simulink model "quad_3_ref_NN"  (R2018b)
settings: Solver=VariableStepAuto  StartTime=0.0  StopTime=20  RelTol=1e-3
undefined symbols (not defined in the file or in its folder): options
libraries: neural x70, simulink x3
(part 2 of 4)

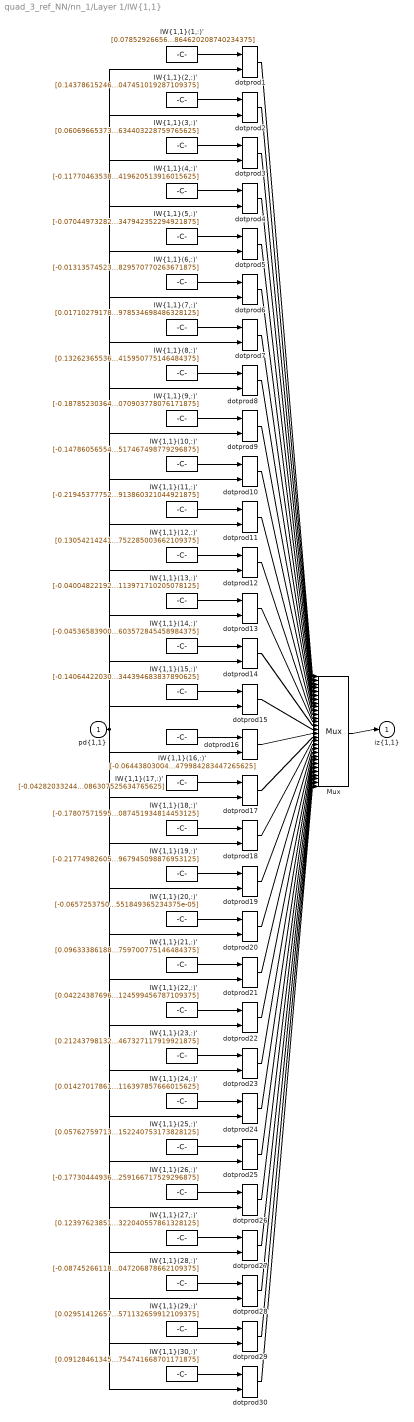
== system quad_3_ref_NN/nn_1/Layer 1/IW{1,1} ==
  "pd{1,1}" : Inport  PortDimensions=12
      mask Display: e = 0.06;c1 = [120 230 180]/255;c2 = ([120 230 180]+0)/(256+128);c3 = ([120 230 180]+128)/(256+128);patch([0 1 1 0],[0 0 1 1],c1);patch([0 1 1 1-e 1-e 0+e],[0 0 1 1-e 0+e 0+e],c2);patch([0 0 1 1-e 0+e 0+e],[0 1 1 1-e 1-e 0+e],c3);plot([0 1 1 0 0],[0 0 1 1 0]);
  "IW{1,1}(1,:)'" : Constant  Value=[0.078529266562737121137871554310549981892108917236328125;0.00786693915550643572964784056011922075413167476654052734375;0.002443768882647874736424586927796553936786949634552001953125;-0.07263690237927265813677735195597051642835140228271484375;0.01107188552850253519810319602356685209088027477264404296875;-0.0207620276565758342390832780210985220037400722503662109375;0.0370645742360258545478046698917751200497150421142578125;0.0256582074103387063057635231189124169759452342987060546875;0.00430276640258473765110469599903808557428419589996337890625;-0.0037272719818124311515206148470724656363017857074737548828125;0.0142728984479785735162149507004869519732892513275146484375;0.01071616499854453029294543142668771906755864620208740234375]
      mask Display: e = 0.06;c1 = [120 150 230]/255;c2 = ([120 150 230]+0)/383;c3 = ([120 150 230]+128)/383;patch([0 1 1 0],[0 0 1 1],c1);patch([0 1 1 1-e 1-e 0+e],[0 0 1 1-e 0+e 0+e],c2);patch([0 0 1 1-e 0+e 0+e],[0 1 1 1-e 1-e 0+e],c3);plot([0 1 1 0 0],[0 0 1 1 0]);disp('Weights');
  "IW{1,1}(10,:)'" : Constant  Value=[-0.147860565541055366534095583119778893887996673583984375;0.0134470182788290378017581616632014629431068897247314453125;-0.0040992668073650852245126685602372162975370883941650390625;0.2037966130921315954793726632487960159778594970703125;-0.02318330531982816522518220381243736483156681060791015625;0.00827620039422155388819657417798225651495158672332763671875;-0.03711045306748207706082354206955642439424991607666015625;-0.010840372744474746635745532330474816262722015380859375;-0.0160737259669415342988596506756948656402528285980224609375;0.005420268773988205779357230085224728100001811981201171875;0.01523382841408883747735814040424884296953678131103515625;0.0193009061476432479398379626900350558571517467498779296875]
      mask Display: e = 0.06;c1 = [120 150 230]/255;c2 = ([120 150 230]+0)/383;c3 = ([120 150 230]+128)/383;patch([0 1 1 0],[0 0 1 1],c1);patch([0 1 1 1-e 1-e 0+e],[0 0 1 1-e 0+e 0+e],c2);patch([0 0 1 1-e 0+e 0+e],[0 1 1 1-e 1-e 0+e],c3);plot([0 1 1 0 0],[0 0 1 1 0]);disp('Weights');
  "IW{1,1}(11,:)'" : Constant  Value=[-0.21945377752996531039997307743760757148265838623046875;0.026810922938275104365768441994077875278890132904052734375;0.0216877503417858934209316856822624686174094676971435546875;0.352460566654302864808556705611408688127994537353515625;0.0480097492404133185939230088479234836995601654052734375;-0.017400965439232397857782785877134301699697971343994140625;-0.134722352421196400751313149157795123755931854248046875;0.028292010630161616713262873190615209750831127166748046875;0.040633554867679867739216348354602814652025699615478515625;0.030043134050046362004682265478550107218325138092041015625;0.03901470178400827382159121725635486654937267303466796875;0.0600659941011620623907418803355540148913860321044921875]
      mask Display: e = 0.06;c1 = [120 150 230]/255;c2 = ([120 150 230]+0)/383;c3 = ([120 150 230]+128)/383;patch([0 1 1 0],[0 0 1 1],c1);patch([0 1 1 1-e 1-e 0+e],[0 0 1 1-e 0+e 0+e],c2);patch([0 0 1 1-e 0+e 0+e],[0 1 1 1-e 1-e 0+e],c3);plot([0 1 1 0 0],[0 0 1 1 0]);disp('Weights');
  "IW{1,1}(12,:)'" : Constant  Value=[0.13054214241561179488115840285900048911571502685546875;-0.010876253958645880348665713199807214550673961639404296875;0.00645744195837419897310294203407465829513967037200927734375;-0.1590334124757807610084370253389352001249790191650390625;0.003502550214369952452653222962908330373466014862060546875;-0.0177574896271106286160801346341031603515148162841796875;0.0307044845016924451697182263387730927206575870513916015625;0.0198496171972888969803339165309807867743074893951416015625;0.0165141943466253805772314677824397222138941287994384765625;-0.008272558443627182900304006807346013374626636505126953125;-0.016577272283062348401383445661849691532552242279052734375;-0.019815470714216541769925328253521001897752285003662109375]
      mask Display: e = 0.06;c1 = [120 150 230]/255;c2 = ([120 150 230]+0)/383;c3 = ([120 150 230]+128)/383;patch([0 1 1 0],[0 0 1 1],c1);patch([0 1 1 1-e 1-e 0+e],[0 0 1 1-e 0+e 0+e],c2);patch([0 0 1 1-e 0+e 0+e],[0 1 1 1-e 1-e 0+e],c3);plot([0 1 1 0 0],[0 0 1 1 0]);disp('Weights');
  "IW{1,1}(13,:)'" : Constant  Value=[-0.0400482219240929915304860742253367789089679718017578125;-0.01136951268733107749120403440201698685996234416961669921875;-0.01275137584911217349115108987689382047392427921295166015625;0.019746638647258070442536137534261797554790973663330078125;-0.0100133008805152988462960905735599226318299770355224609375;0.00554886997693828688815731453587432042695581912994384765625;-0.0207279164856813795381196285916303168050944805145263671875;-0.0132145956485405884073269788814286584965884685516357421875;-0.0154206941241152480082110542980444733984768390655517578125;-0.0017440958504595879298426641668129377649165689945220947265625;-0.0118417785038119893759045453407452441751956939697265625;-0.0003297525368371159899816280614004426752217113971710205078125]
      mask Display: e = 0.06;c1 = [120 150 230]/255;c2 = ([120 150 230]+0)/383;c3 = ([120 150 230]+128)/383;patch([0 1 1 0],[0 0 1 1],c1);patch([0 1 1 1-e 1-e 0+e],[0 0 1 1-e 0+e 0+e],c2);patch([0 0 1 1-e 0+e 0+e],[0 1 1 1-e 1-e 0+e],c3);plot([0 1 1 0 0],[0 0 1 1 0]);disp('Weights');
  "IW{1,1}(14,:)'" : Constant  Value=[-0.04536583900623207543656434381773578934371471405029296875;0.015322325707905641578587818685264210216701030731201171875;0.016285107900788527157676099932359647937119007110595703125;0.01209169860414867347930822916168835945427417755126953125;-0.009840496063433755435934102706596604548394680023193359375;-0.001097090523768812393712313024707327713258564472198486328125;0.00288142231145414873250132359316921792924404144287109375;0.000899839764804431958833408344844428938813507556915283203125;-0.00132219817163032292428592739952364354394376277923583984375;0.01485548166720073066937590766656285268254578113555908203125;0.00875988621009281265283874517990625463426113128662109375;0.00159143009482582385716309403278501122258603572845458984375]
      mask Display: e = 0.06;c1 = [120 150 230]/255;c2 = ([120 150 230]+0)/383;c3 = ([120 150 230]+128)/383;patch([0 1 1 0],[0 0 1 1],c1);patch([0 1 1 1-e 1-e 0+e],[0 0 1 1-e 0+e 0+e],c2);patch([0 0 1 1-e 0+e 0+e],[0 1 1 1-e 1-e 0+e],c3);plot([0 1 1 0 0],[0 0 1 1 0]);disp('Weights');
  "IW{1,1}(15,:)'" : Constant  Value=[-0.1406442203035578042413789034981164149940013885498046875;-0.00489135033403387264883122043102048337459564208984375;-0.003944791983629051916604435490398827823810279369354248046875;0.1445432054926384657367322006393806077539920806884765625;-0.0130691593280128637299952742978348396718502044677734375;0.01510921933796705897423695574843804934062063694000244140625;-0.08150926462194003907502093397852149792015552520751953125;0.00943571383983794580163628751279247808270156383514404296875;0.01004127751787367399394224065645175869576632976531982421875;-0.0183353986201333536698587778346336563117802143096923828125;-0.0157985391490613018283806212593844975344836711883544921875;-0.0161584671239796452690828942877487861551344394683837890625]
      mask Display: e = 0.06;c1 = [120 150 230]/255;c2 = ([120 150 230]+0)/383;c3 = ([120 150 230]+128)/383;patch([0 1 1 0],[0 0 1 1],c1);patch([0 1 1 1-e 1-e 0+e],[0 0 1 1-e 0+e 0+e],c2);patch([0 0 1 1-e 0+e 0+e],[0 1 1 1-e 1-e 0+e],c3);plot([0 1 1 0 0],[0 0 1 1 0]);disp('Weights');
  "IW{1,1}(16,:)'" : Constant  Value=[-0.0644380300412848161517587186608579941093921661376953125;0.001197491485301433768173584581973045715130865573883056640625;-0.002973574198419578172580823860471355146728456020355224609375;0.07261552598673505498627633869546116329729557037353515625;-0.00911983882616861606107416804434251389466226100921630859375;0.002258921289302671768506325378211840870790183544158935546875;-0.01497592283162310113076021167444196180440485477447509765625;0.00432259258477654152719171776197981671430170536041259765625;-0.01530863786152473517143679515584153705276548862457275390625;0.0011924005049313009078904013193778155255131423473358154296875;0.001075716311985324726008261819742983789183199405670166015625;-0.0180167069664866098810396266571842716075479984283447265625]
      mask Display: e = 0.06;c1 = [120 150 230]/255;c2 = ([120 150 230]+0)/383;c3 = ([120 150 230]+128)/383;patch([0 1 1 0],[0 0 1 1],c1);patch([0 1 1 1-e 1-e 0+e],[0 0 1 1-e 0+e 0+e],c2);patch([0 0 1 1-e 0+e 0+e],[0 1 1 1-e 1-e 0+e],c3);plot([0 1 1 0 0],[0 0 1 1 0]);disp('Weights');
  "IW{1,1}(17,:)'" : Constant  Value=[-0.042820332449136418173640805662216735072433948516845703125;-0.0065443141325867669466642695397240458987653255462646484375;-0.01513063676343030621029850379954950767569243907928466796875;0.032196066510549424533049744923118851147592067718505859375;-0.0033468345050003613268263524815893106278963387012481689453125;0.00461329995651396131128851862968076602555811405181884765625;-0.002691478208598889650116081639907861244864761829376220703125;0.000650547080040542353984722723225786467082798480987548828125;-0.01729420381033273945714512365157133899629116058349609375;0.00405337807023969064201818213177830330096185207366943359375;-0.01149323371723583175896266084237140603363513946533203125;-0.0045561415204842282966612998507116572000086307525634765625]
      mask Display: e = 0.06;c1 = [120 150 230]/255;c2 = ([120 150 230]+0)/383;c3 = ([120 150 230]+128)/383;patch([0 1 1 0],[0 0 1 1],c1);patch([0 1 1 1-e 1-e 0+e],[0 0 1 1-e 0+e 0+e],c2);patch([0 0 1 1-e 0+e 0+e],[0 1 1 1-e 1-e 0+e],c3);plot([0 1 1 0 0],[0 0 1 1 0]);disp('Weights');
  "IW{1,1}(18,:)'" : Constant  Value=[-0.1780757159575738768353403429500758647918701171875;-0.019521046281996905225053495769316214136779308319091796875;-0.02148481740437359344131351690521114505827426910400390625;0.2394798892014605995459675114034325815737247467041015625;0.020440374862543873868414578964802785776555538177490234375;-0.01235558398060544217644807218903224566020071506500244140625;-0.1228380733929725909803210015525110065937042236328125;0.0139497234295006093673929825627055834047496318817138671875;0.01213816245689446071676087512969388626515865325927734375;-0.033165603622792076687897377951230737380683422088623046875;-0.0269775987766404691525767844950678409077227115631103515625;-0.0084178593815306575198764704737186548300087451934814453125]
      mask Display: e = 0.06;c1 = [120 150 230]/255;c2 = ([120 150 230]+0)/383;c3 = ([120 150 230]+128)/383;patch([0 1 1 0],[0 0 1 1],c1);patch([0 1 1 1-e 1-e 0+e],[0 0 1 1-e 0+e 0+e],c2);patch([0 0 1 1-e 0+e 0+e],[0 1 1 1-e 1-e 0+e],c3);plot([0 1 1 0 0],[0 0 1 1 0]);disp('Weights');
  "IW{1,1}(19,:)'" : Constant  Value=[-0.2177498260504428240214025436216616071760654449462890625;0.0185045242913031461606809813247309648431837558746337890625;0.0016690905058854392517542208906888845376670360565185546875;0.25350570394707194754602141983923502266407012939453125;0.0080543188283483217737579451522833551280200481414794921875;-0.003408997157735411953627391312693362124264240264892578125;-0.1300658296282164172463780005273292772471904754638671875;0.0118027299680211437971077970132682821713387966156005859375;-0.009127017617710224406391006368721718899905681610107421875;0.00992258872258855451065073793870396912097930908203125;-0.000647670814953184292850352221648790873587131500244140625;-0.012919553810417212791339380828503635711967945098876953125]
      mask Display: e = 0.06;c1 = [120 150 230]/255;c2 = ([120 150 230]+0)/383;c3 = ([120 150 230]+128)/383;patch([0 1 1 0],[0 0 1 1],c1);patch([0 1 1 1-e 1-e 0+e],[0 0 1 1-e 0+e 0+e],c2);patch([0 0 1 1-e 0+e 0+e],[0 1 1 1-e 1-e 0+e],c3);plot([0 1 1 0 0],[0 0 1 1 0]);disp('Weights');
  "IW{1,1}(2,:)'" : Constant  Value=[0.1437861524654724387772830596077255904674530029296875;-0.004658330850192315443492052651208723546005785465240478515625;0.0166751004439475158935834997464553453028202056884765625;-0.163922574492781636390503763323067687451839447021484375;0.01526933862748157400002213535117334686219692230224609375;-0.00976544107933535916743483795698921312578022480010986328125;0.054240136556781330667842411230594734661281108856201171875;0.013842710387504543467773743259385810233652591705322265625;0.008788677192960343831362735045331646688282489776611328125;0.0143984192110828169985925484297695220448076725006103515625;0.02277789638211417944102521460081334225833415985107421875;0.018991406808802978323225119083872414194047451019287109375]
      mask Display: e = 0.06;c1 = [120 150 230]/255;c2 = ([120 150 230]+0)/383;c3 = ([120 150 230]+128)/383;patch([0 1 1 0],[0 0 1 1],c1);patch([0 1 1 1-e 1-e 0+e],[0 0 1 1-e 0+e 0+e],c2);patch([0 0 1 1-e 0+e 0+e],[0 1 1 1-e 1-e 0+e],c3);plot([0 1 1 0 0],[0 0 1 1 0]);disp('Weights');
  "IW{1,1}(20,:)'" : Constant  Value=[-0.06572537506185331668273619243336725048720836639404296875;0.01669642639971923026021016767117544077336788177490234375;0.01438697051899651656314826908555914997123181819915771484375;0.097990860021580694638743125324253924190998077392578125;-0.023250392969835768919306673296887311153113842010498046875;0.034191678885905997520300303449403145350515842437744140625;0.00207157777178058714884212321294398861937224864959716796875;-0.03102709202383165110195051283881184644997119903564453125;-0.02967893733167838166142615818898775614798069000244140625;0.01480263260132471010710464298654187587089836597442626953125;0.0152700053015788032861888012803319725207984447479248046875;-3.5242403931787756599103289545382722280919551849365234375e-05]
      mask Display: e = 0.06;c1 = [120 150 230]/255;c2 = ([120 150 230]+0)/383;c3 = ([120 150 230]+128)/383;patch([0 1 1 0],[0 0 1 1],c1);patch([0 1 1 1-e 1-e 0+e],[0 0 1 1-e 0+e 0+e],c2);patch([0 0 1 1-e 0+e 0+e],[0 1 1 1-e 1-e 0+e],c3);plot([0 1 1 0 0],[0 0 1 1 0]);disp('Weights');
  "IW{1,1}(21,:)'" : Constant  Value=[0.0963338618860876960692252168882987461984157562255859375;-0.017399790836133639804206296730626490898430347442626953125;-0.0190305406288347016274808964908515918068587779998779296875;-0.08916389166021602974421256249115685932338237762451171875;0.00790176839013517588738988450813849340192973613739013671875;-0.01478596274658084720743378426277558901347219944000244140625;0.0029569260110624100146292647650625440292060375213623046875;0.02925230114780884294045648630344658158719539642333984375;0.01150080739869995503921185076023903093300759792327880859375;-0.0173239132576814454378411056723052752204239368438720703125;-0.0251577527719447739673608310795316356234252452850341796875;-0.0284567136595101910501171005307696759700775146484375]
      mask Display: e = 0.06;c1 = [120 150 230]/255;c2 = ([120 150 230]+0)/383;c3 = ([120 150 230]+128)/383;patch([0 1 1 0],[0 0 1 1],c1);patch([0 1 1 1-e 1-e 0+e],[0 0 1 1-e 0+e 0+e],c2);patch([0 0 1 1-e 0+e 0+e],[0 1 1 1-e 1-e 0+e],c3);plot([0 1 1 0 0],[0 0 1 1 0]);disp('Weights');
  "IW{1,1}(22,:)'" : Constant  Value=[0.04224387696688165771963241468256455846130847930908203125;-0.0072788809324365842667869941351455054245889186859130859375;-0.00776694166044583807206880265994186629541218280792236328125;-0.039942992962429001158053409881176776252686977386474609375;-0.002529471782466141509260193487307333271019160747528076171875;2.276536562523766293875127075807540677487850189208984375e-05;0.004836203064547402001582820929570516454987227916717529296875;-0.00802404233775699630981659282724649528972804546356201171875;-0.0010166811297409139407121880793738455395214259624481201171875;-0.0021571010148963682372114103458216050057671964168548583984375;0.005758936473604313842356017261181477806530892848968505859375;-0.0109210797386651535523238720770677900873124599456787109375]
      mask Display: e = 0.06;c1 = [120 150 230]/255;c2 = ([120 150 230]+0)/383;c3 = ([120 150 230]+128)/383;patch([0 1 1 0],[0 0 1 1],c1);patch([0 1 1 1-e 1-e 0+e],[0 0 1 1-e 0+e 0+e],c2);patch([0 0 1 1-e 0+e 0+e],[0 1 1 1-e 1-e 0+e],c3);plot([0 1 1 0 0],[0 0 1 1 0]);disp('Weights');
  "IW{1,1}(23,:)'" : Constant  Value=[0.2124379813207072087433147089541307650506496429443359375;0.0271084126562651517300395198617479763925075531005859375;0.03617241440309056088597827738340129144489765167236328125;-0.2329129512256800371705622865192708559334278106689453125;-0.006326850035338311452337567430959097691811621189117431640625;0.007198988072314660251194151641129792551510035991668701171875;0.138206806871398246716609037321177311241626739501953125;-0.0061215828864918837848296817583104711957275867462158203125;-0.01262176943427284481202832466806285083293914794921875;0.024705513504592720164243502267709118314087390899658203125;0.0263874965393726020057574288557589170522987842559814453125;0.03807250938564780973205614600374246947467327117919921875]
      mask Display: e = 0.06;c1 = [120 150 230]/255;c2 = ([120 150 230]+0)/383;c3 = ([120 150 230]+128)/383;patch([0 1 1 0],[0 0 1 1],c1);patch([0 1 1 1-e 1-e 0+e],[0 0 1 1-e 0+e 0+e],c2);patch([0 0 1 1-e 0+e 0+e],[0 1 1 1-e 1-e 0+e],c3);plot([0 1 1 0 0],[0 0 1 1 0]);disp('Weights');
  "IW{1,1}(24,:)'" : Constant  Value=[0.01427017861859124214785055073662078939378261566162109375;-0.00599730328078098597066603048233446315862238407135009765625;-0.00229647485082267073519535216519216191954910755157470703125;-0.004921686700011855541969651994804735295474529266357421875;0.0033036694095360864299737446714289035298861563205718994140625;-0.0116597984915904999414504317201135563664138317108154296875;0.005306498758002420150503564144628398935310542583465576171875;0.02005055165372159053926992555716424249112606048583984375;0.0162077445173333702099771613802658976055681705474853515625;-0.0045361261791746036731165503397278371267020702362060546875;0.00656465040648158450198312863221872248686850070953369140625;0.01683363396966587599568043742692680098116397857666015625]
      mask Display: e = 0.06;c1 = [120 150 230]/255;c2 = ([120 150 230]+0)/383;c3 = ([120 150 230]+128)/383;patch([0 1 1 0],[0 0 1 1],c1);patch([0 1 1 1-e 1-e 0+e],[0 0 1 1-e 0+e 0+e],c2);patch([0 0 1 1-e 0+e 0+e],[0 1 1 1-e 1-e 0+e],c3);plot([0 1 1 0 0],[0 0 1 1 0]);disp('Weights');
  "IW{1,1}(25,:)'" : Constant  Value=[0.05762759713787439508347887340278248302638530731201171875;0.00569852081166601596995402445600120699964463710784912109375;-0.0100954629227731629281805680875550024211406707763671875;-0.038802111759898283427361320718773640692234039306640625;0.01723594123708850622822552622892544604837894439697265625;-0.015320391135778550772972295135332387872040271759033203125;-0.0048072586970143056650517365824271109886467456817626953125;0.018245931899519472751958204526090412400662899017333984375;0.01915020901981535905722608958967612124979496002197265625;-0.00139635998883026464338630301398325173067860305309295654296875;-0.004723050154852247682624177826937739155255258083343505859375;0.003040463749679207794418545063308556564152240753173828125]
      mask Display: e = 0.06;c1 = [120 150 230]/255;c2 = ([120 150 230]+0)/383;c3 = ([120 150 230]+128)/383;patch([0 1 1 0],[0 0 1 1],c1);patch([0 1 1 1-e 1-e 0+e],[0 0 1 1-e 0+e 0+e],c2);patch([0 0 1 1-e 0+e 0+e],[0 1 1 1-e 1-e 0+e],c3);plot([0 1 1 0 0],[0 0 1 1 0]);disp('Weights');
  "IW{1,1}(26,:)'" : Constant  Value=[-0.1773044493602602134085799434615182690322399139404296875;-0.01174161297476089375890762056542371283285319805145263671875;0.00254904182041163114569304326550991390831768512725830078125;0.248063223573464830540302727968082763254642486572265625;0.00975418781999848848174305970815112232230603694915771484375;-0.0032034856226173329639406173185989246121607720851898193359375;-0.09679320201552164826264146313405944965779781341552734375;0.0158327200921912492059817623157869093120098114013671875;0.024295591623219724153326382065642974339425563812255859375;0.005290875181447407017698569831054555834271013736724853515625;-0.0037320284637027494566152707733408533385954797267913818359375;-0.0054249659038856472281775467081388342194259166717529296875]
      mask Display: e = 0.06;c1 = [120 150 230]/255;c2 = ([120 150 230]+0)/383;c3 = ([120 150 230]+128)/383;patch([0 1 1 0],[0 0 1 1],c1);patch([0 1 1 1-e 1-e 0+e],[0 0 1 1-e 0+e 0+e],c2);patch([0 0 1 1-e 0+e 0+e],[0 1 1 1-e 1-e 0+e],c3);plot([0 1 1 0 0],[0 0 1 1 0]);disp('Weights');
  "IW{1,1}(27,:)'" : Constant  Value=[0.12397623851760118662834742053746595047414302825927734375;0.00703020509924084761876894589249786804430186748504638671875;-0.0088155685346204444574613745544411358423531055450439453125;-0.14936136269416733224346671704552136361598968505859375;0.011564624200221473859784282467444427311420440673828125;-0.0073422551095141154464673860502443858422338962554931640625;0.0380891805065197985857849971580435521900653839111328125;0.0129839175273246364150647735868915333412587642669677734375;0.00534807313427830034735510622567744576372206211090087890625;-0.0106017759053239346567210077409981749951839447021484375;0.002154003700883188980597093831192978541366755962371826171875;0.004948994620806485174313582575678083230741322040557861328125]
      mask Display: e = 0.06;c1 = [120 150 230]/255;c2 = ([120 150 230]+0)/383;c3 = ([120 150 230]+128)/383;patch([0 1 1 0],[0 0 1 1],c1);patch([0 1 1 1-e 1-e 0+e],[0 0 1 1-e 0+e 0+e],c2);patch([0 0 1 1-e 0+e 0+e],[0 1 1 1-e 1-e 0+e],c3);plot([0 1 1 0 0],[0 0 1 1 0]);disp('Weights');
  "IW{1,1}(28,:)'" : Constant  Value=[-0.0874526611894194394469792541713104583323001861572265625;0.00835174689493858694866457170746798510663211345672607421875;0.0080794051668903014984390864583474467508494853973388671875;0.09048192418525609348467497738965903408825397491455078125;-0.015356527752780339823868160920028458349406719207763671875;0.01306441571321059931520824903827815433032810688018798828125;-0.01743385658574313212820783292045234702527523040771484375;-0.015506033913388637957009308365741162560880184173583984375;-0.001906468197211591379669481938208264182321727275848388671875;0.00966799630999645547013710000783248688094317913055419921875;0.0113713020500187216021981129188134218566119670867919921875;0.003546484887744518442465047058931304491125047206878662109375]
      mask Display: e = 0.06;c1 = [120 150 230]/255;c2 = ([120 150 230]+0)/383;c3 = ([120 150 230]+128)/383;patch([0 1 1 0],[0 0 1 1],c1);patch([0 1 1 1-e 1-e 0+e],[0 0 1 1-e 0+e 0+e],c2);patch([0 0 1 1-e 0+e 0+e],[0 1 1 1-e 1-e 0+e],c3);plot([0 1 1 0 0],[0 0 1 1 0]);disp('Weights');
  "IW{1,1}(29,:)'" : Constant  Value=[0.0295141265783554866686255735430677304975688457489013671875;-0.0070460519595088137723148946633955347351729869842529296875;0.001857410501974206436248682194900538888759911060333251953125;-0.0271064656877724081962544033785889041610062122344970703125;0.0149766443193747079976052560823518433608114719390869140625;-0.005566702202152033589210855524243015679530799388885498046875;-0.0055767540223188548365040873022735468111932277679443359375;0.002347103935738591336257474750937035423703491687774658203125;-0.0007824621553606009478898375419930744101293385028839111328125;-0.0096625590261764406074806998958592885173857212066650390625;0.003723223284914132548417686763286837958730757236480712890625;0.0126047283902711304559574045924819074571132659912109375]
      mask Display: e = 0.06;c1 = [120 150 230]/255;c2 = ([120 150 230]+0)/383;c3 = ([120 150 230]+128)/383;patch([0 1 1 0],[0 0 1 1],c1);patch([0 1 1 1-e 1-e 0+e],[0 0 1 1-e 0+e 0+e],c2);patch([0 0 1 1-e 0+e 0+e],[0 1 1 1-e 1-e 0+e],c3);plot([0 1 1 0 0],[0 0 1 1 0]);disp('Weights');
  "IW{1,1}(3,:)'" : Constant  Value=[0.060696653730429629691744963793098577298223972320556640625;-0.015937068522683332794098731710619176737964153289794921875;-0.01240571554046476961119527260279937763698399066925048828125;-0.0274290427605467686256179860038173501379787921905517578125;-0.0004568232106143717274893134572266717441380023956298828125;-0.006669316018269409208907294583923430764116346836090087890625;0.0042327149496002892947732476613964536227285861968994140625;0.02097878949725838493289842290323576889932155609130859375;0.007579927949637425312057192883230527513660490512847900390625;-0.0198344679543810652189161913838688633404672145843505859375;-0.017550425617539271161415825872609275393187999725341796875;-0.0149397170245573231162072858069223002530634403228759765625]
      mask Display: e = 0.06;c1 = [120 150 230]/255;c2 = ([120 150 230]+0)/383;c3 = ([120 150 230]+128)/383;patch([0 1 1 0],[0 0 1 1],c1);patch([0 1 1 1-e 1-e 0+e],[0 0 1 1-e 0+e 0+e],c2);patch([0 0 1 1-e 0+e 0+e],[0 1 1 1-e 1-e 0+e],c3);plot([0 1 1 0 0],[0 0 1 1 0]);disp('Weights');
  "IW{1,1}(30,:)'" : Constant  Value=[0.0912846134508133733032053669376182369887828826904296875;0.01138731321142053519446246667712330236099660396575927734375;-0.004424901047140802727575259467585055972449481487274169921875;-0.10131814151688796343808718347645481117069721221923828125;0.000152514314671614581442327107652090489864349365234375;-0.0199830302233286079272023272324076970107853412628173828125;0.036897676355063746544971081675612367689609527587890625;0.005003935723600807898570064224941233987919986248016357421875;-0.003743298228545082102780572341771403443999588489532470703125;-0.004154480549329501483379889492653092020191252231597900390625;0.01332716682037082649159298597396627883426845073699951171875;0.0060988865869046997303382084965051035396754741668701171875]
      mask Display: e = 0.06;c1 = [120 150 230]/255;c2 = ([120 150 230]+0)/383;c3 = ([120 150 230]+128)/383;patch([0 1 1 0],[0 0 1 1],c1);patch([0 1 1 1-e 1-e 0+e],[0 0 1 1-e 0+e 0+e],c2);patch([0 0 1 1-e 0+e 0+e],[0 1 1 1-e 1-e 0+e],c3);plot([0 1 1 0 0],[0 0 1 1 0]);disp('Weights');
  "IW{1,1}(4,:)'" : Constant  Value=[-0.1177046353856912308533111399810877628624439239501953125;0.001125346529822400520881586771793081425130367279052734375;-0.005657217312278520725266073299053459777496755123138427734375;0.1078803885504474868728408409879193641245365142822265625;-0.0069362270758731338349267758758287527598440647125244140625;0.02058494455196889505455004609757452271878719329833984375;-0.0300000263414266395145535426536298473365604877471923828125;-0.00633278730361327459041920207027942524291574954986572265625;-0.0002339706542385071308398636347192223183810710906982421875;-0.0113163105219613140117740357482034596614539623260498046875;-0.03340003359113496994581282706349156796932220458984375;-0.031610446291984541089536975277951569296419620513916015625]
      mask Display: e = 0.06;c1 = [120 150 230]/255;c2 = ([120 150 230]+0)/383;c3 = ([120 150 230]+128)/383;patch([0 1 1 0],[0 0 1 1],c1);patch([0 1 1 1-e 1-e 0+e],[0 0 1 1-e 0+e 0+e],c2);patch([0 0 1 1-e 0+e 0+e],[0 1 1 1-e 1-e 0+e],c3);plot([0 1 1 0 0],[0 0 1 1 0]);disp('Weights');
  "IW{1,1}(5,:)'" : Constant  Value=[-0.0704497328258970878511746604999643750488758087158203125;-0.00943083781139679271088294143510211142711341381072998046875;-0.0090738792430153265844428034370139357633888721466064453125;0.06312132545929947935459125574197969399392604827880859375;-0.020785357775132733137990470595468650572001934051513671875;0.0133348500938768425860825317386115784756839275360107421875;-0.0352948156836478676989798941576736979186534881591796875;-0.0157145869916970049029458778022672049701213836669921875;-0.02184810102009000776224212359011289663612842559814453125;0.0018370058675048713849042858470284045324660837650299072265625;-0.0046927518855038284628644618123871623538434505462646484375;-0.00291307609302979102217090456861114944331347942352294921875]
      mask Display: e = 0.06;c1 = [120 150 230]/255;c2 = ([120 150 230]+0)/383;c3 = ([120 150 230]+128)/383;patch([0 1 1 0],[0 0 1 1],c1);patch([0 1 1 1-e 1-e 0+e],[0 0 1 1-e 0+e 0+e],c2);patch([0 0 1 1-e 0+e 0+e],[0 1 1 1-e 1-e 0+e],c3);plot([0 1 1 0 0],[0 0 1 1 0]);disp('Weights');
  "IW{1,1}(6,:)'" : Constant  Value=[-0.0131357452396844189002056424442343995906412601470947265625;-0.0028033225603488151102260506064567380235530436038970947265625;0.0140067287639270114663059274562328937463462352752685546875;0.0295771484731742508034191274646218516863882541656494140625;-0.0001520422418176225858033046023365386645309627056121826171875;0.01252984203624300275914382751807352178730070590972900390625;-0.015315558031886646050967470955583848990499973297119140625;0.016461816979809980321380891155058634467422962188720703125;0.01007792572858965361726202303316313191317021846771240234375;-0.005045751469591740721865047447636243305169045925140380859375;-0.006010718906724117627238257455246639437973499298095703125;-0.00225202291983665758845489790473948232829570770263671875]
      mask Display: e = 0.06;c1 = [120 150 230]/255;c2 = ([120 150 230]+0)/383;c3 = ([120 150 230]+128)/383;patch([0 1 1 0],[0 0 1 1],c1);patch([0 1 1 1-e 1-e 0+e],[0 0 1 1-e 0+e 0+e],c2);patch([0 0 1 1-e 0+e 0+e],[0 1 1 1-e 1-e 0+e],c3);plot([0 1 1 0 0],[0 0 1 1 0]);disp('Weights');
  "IW{1,1}(7,:)'" : Constant  Value=[0.0171027917807706590636040999697797815315425395965576171875;0.013089396728321885110535305329904076643288135528564453125;0.00789126491498782882405560457073079305700957775115966796875;-0.00548230330131020682227216411774861626327037811279296875;-0.0085804763815275318650233060679966001771390438079833984375;0.00918476027664482698453785047831843257881700992584228515625;0.0085532010392050210334513593579686130397021770477294921875;0.003718651007595575978814661510796213406138122081756591796875;0.00624996195524041113500413047177062253467738628387451171875;0.0116131380822985623424425938310378114692866802215576171875;0.0090118921456736507391571677771935355849564075469970703125;0.00538541488834482114100854488469849457032978534698486328125]
      mask Display: e = 0.06;c1 = [120 150 230]/255;c2 = ([120 150 230]+0)/383;c3 = ([120 150 230]+128)/383;patch([0 1 1 0],[0 0 1 1],c1);patch([0 1 1 1-e 1-e 0+e],[0 0 1 1-e 0+e 0+e],c2);patch([0 0 1 1-e 0+e 0+e],[0 1 1 1-e 1-e 0+e],c3);plot([0 1 1 0 0],[0 0 1 1 0]);disp('Weights');
  "IW{1,1}(8,:)'" : Constant  Value=[0.1326236553670202267252165029276511631906032562255859375;-0.0105686609151273980256036111313733272254467010498046875;0.00421792029094246456732975047998479567468166351318359375;-0.15042769984248760550826773396693170070648193359375;0.0031045123121772448017419154808749226504005491733551025390625;-0.0072963541966421692486211014738728408701717853546142578125;0.067665644951662662354152644184068776667118072509765625;-0.000537408071939224178670269083113453234545886516571044921875;0.002607573073016599025930606359224839252419769763946533203125;0.0067980713737081609193690923120811930857598781585693359375;0.006825841974759887416379644520247893524356186389923095703125;0.0027036554837576685927924557972801267169415950775146484375]
      mask Display: e = 0.06;c1 = [120 150 230]/255;c2 = ([120 150 230]+0)/383;c3 = ([120 150 230]+128)/383;patch([0 1 1 0],[0 0 1 1],c1);patch([0 1 1 1-e 1-e 0+e],[0 0 1 1-e 0+e 0+e],c2);patch([0 0 1 1-e 0+e 0+e],[0 1 1 1-e 1-e 0+e],c3);plot([0 1 1 0 0],[0 0 1 1 0]);disp('Weights');
  "IW{1,1}(9,:)'" : Constant  Value=[-0.187852303647385532325841950296307913959026336669921875;0.00775085827047730484273824203000913257710635662078857421875;-0.00444039105421620804159399398258756264112889766693115234375;0.260207055625680194754778540300321765244007110595703125;-0.001153947157839335137252678720187759608961641788482666015625;0.011968407457842229757449814542269450612366199493408203125;-0.08117185044082531053533102749497629702091217041015625;0.006046974828518562015966519851417615427635610103607177734375;0.0110136827995899987120420604469472891651093959808349609375;0.013686626702872177474556991683130036108195781707763671875;0.02338955771501345648477609984183800406754016876220703125;0.013221189598115405672285049831771175377070903778076171875]
      mask Display: e = 0.06;c1 = [120 150 230]/255;c2 = ([120 150 230]+0)/383;c3 = ([120 150 230]+128)/383;patch([0 1 1 0],[0 0 1 1],c1);patch([0 1 1 1-e 1-e 0+e],[0 0 1 1-e 0+e 0+e],c2);patch([0 0 1 1-e 0+e 0+e],[0 1 1 1-e 1-e 0+e],c3);plot([0 1 1 0 0],[0 0 1 1 0]);disp('Weights');
  Mux : Mux  Inputs=30
      mask Display: e = 0.06;c1 = [120 150 230]/255;c2 = ([120 150 230]+0)/383;c3 = ([120 150 230]+128)/383;patch([0 1 1 0],[0 0 1 1],c1);patch([0 1 1 1-e 1-e 0+e],[0 0 1 1-e 0+e 0+e],c2);patch([0 0 1 1-e 0+e 0+e],[0 1 1 1-e 1-e 0+e],c3);plot([0 1 1 0 0],[0 0 1 1 0]);disp('Mux');
  dotprod{1..30} (30 alike) : neural/Weight Functions/dotprod
  "iz{1,1}" : Outport
      mask Display: e = 0.06;c1 = [120 230 180]/255;c2 = ([120 230 180]+0)/(256+128);c3 = ([120 230 180]+128)/(256+128);patch([0 1 1 0],[0 0 1 1],c1);patch([0 1 1 1-e 1-e 0+e],[0 0 1 1-e 0+e 0+e],c2);patch([0 0 1 1-e 0+e 0+e],[0 1 1 1-e 1-e 0+e],c3);plot([0 1 1 0 0],[0 0 1 1 0]);
  wires:
  "IW{1,1}(1,:)'"/1 -> dotprod1/1
  "pd{1,1}"/1 -> dotprod1/2, dotprod2/2, dotprod3/2, dotprod4/2, dotprod5/2, dotprod6/2, dotprod7/2, dotprod8/2, dotprod9/2, dotprod10/2, dotprod11/2, dotprod12/2, dotprod13/2, dotprod14/2, dotprod15/2, dotprod16/2, dotprod17/2, dotprod18/2, dotprod19/2, dotprod20/2, dotprod21/2, dotprod22/2, dotprod23/2, dotprod24/2, dotprod25/2, dotprod26/2, dotprod27/2, dotprod28/2, dotprod29/2, dotprod30/2
  dotprod1/1 -> Mux/1
  "IW{1,1}(2,:)'"/1 -> dotprod2/1
  dotprod2/1 -> Mux/2
  "IW{1,1}(3,:)'"/1 -> dotprod3/1
  dotprod3/1 -> Mux/3
  "IW{1,1}(4,:)'"/1 -> dotprod4/1
  dotprod4/1 -> Mux/4
  "IW{1,1}(5,:)'"/1 -> dotprod5/1
  dotprod5/1 -> Mux/5
  "IW{1,1}(6,:)'"/1 -> dotprod6/1
  dotprod6/1 -> Mux/6
  "IW{1,1}(7,:)'"/1 -> dotprod7/1
  dotprod7/1 -> Mux/7
  "IW{1,1}(8,:)'"/1 -> dotprod8/1
  dotprod8/1 -> Mux/8
  "IW{1,1}(9,:)'"/1 -> dotprod9/1
  dotprod9/1 -> Mux/9
  "IW{1,1}(10,:)'"/1 -> dotprod10/1
  dotprod10/1 -> Mux/10
  "IW{1,1}(11,:)'"/1 -> dotprod11/1
  dotprod11/1 -> Mux/11
  "IW{1,1}(12,:)'"/1 -> dotprod12/1
  dotprod12/1 -> Mux/12
  "IW{1,1}(13,:)'"/1 -> dotprod13/1
  dotprod13/1 -> Mux/13
  "IW{1,1}(14,:)'"/1 -> dotprod14/1
  dotprod14/1 -> Mux/14
  "IW{1,1}(15,:)'"/1 -> dotprod15/1
  dotprod15/1 -> Mux/15
  "IW{1,1}(16,:)'"/1 -> dotprod16/1
  dotprod16/1 -> Mux/16
  "IW{1,1}(17,:)'"/1 -> dotprod17/1
  dotprod17/1 -> Mux/17
  "IW{1,1}(18,:)'"/1 -> dotprod18/1
  dotprod18/1 -> Mux/18
  "IW{1,1}(19,:)'"/1 -> dotprod19/1
  dotprod19/1 -> Mux/19
  "IW{1,1}(20,:)'"/1 -> dotprod20/1
  dotprod20/1 -> Mux/20
  "IW{1,1}(21,:)'"/1 -> dotprod21/1
  dotprod21/1 -> Mux/21
  "IW{1,1}(22,:)'"/1 -> dotprod22/1
  dotprod22/1 -> Mux/22
  "IW{1,1}(23,:)'"/1 -> dotprod23/1
  dotprod23/1 -> Mux/23
  "IW{1,1}(24,:)'"/1 -> dotprod24/1
  dotprod24/1 -> Mux/24
  "IW{1,1}(25,:)'"/1 -> dotprod25/1
  dotprod25/1 -> Mux/25
  "IW{1,1}(26,:)'"/1 -> dotprod26/1
  dotprod26/1 -> Mux/26
  "IW{1,1}(27,:)'"/1 -> dotprod27/1
  dotprod27/1 -> Mux/27
  "IW{1,1}(28,:)'"/1 -> dotprod28/1
  dotprod28/1 -> Mux/28
  "IW{1,1}(29,:)'"/1 -> dotprod29/1
  dotprod29/1 -> Mux/29
  "IW{1,1}(30,:)'"/1 -> dotprod30/1
  dotprod30/1 -> Mux/30
  Mux/1 -> "iz{1,1}"/1

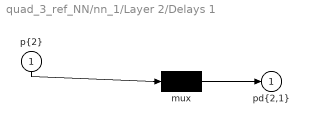
== system quad_3_ref_NN/nn_1/Layer 2/Delays 1 ==
  "p{2}" : Inport  PortDimensions=30
      mask Display: e = 0.06;c1 = [120 230 180]/255;c2 = ([120 230 180]+0)/(256+128);c3 = ([120 230 180]+128)/(256+128);patch([0 1 1 0],[0 0 1 1],c1);patch([0 1 1 1-e 1-e 0+e],[0 0 1 1-e 0+e 0+e],c2);patch([0 0 1 1-e 0+e 0+e],[0 1 1 1-e 1-e 0+e],c3);plot([0 1 1 0 0],[0 0 1 1 0]);
  mux : Mux  Inputs=1
      mask Display: e = 0.06;c1 = [120 150 230]/255;c2 = ([120 150 230]+0)/383;c3 = ([120 150 230]+128)/383;patch([0 1 1 0],[0 0 1 1],c1);patch([0 1 1 1-e 1-e 0+e],[0 0 1 1-e 0+e 0+e],c2);patch([0 0 1 1-e 0+e 0+e],[0 1 1 1-e 1-e 0+e],c3);plot([0 1 1 0 0],[0 0 1 1 0]);disp('Mux')
  "pd{2,1}" : Outport
      mask Display: e = 0.06;c1 = [120 230 180]/255;c2 = ([120 230 180]+0)/(256+128);c3 = ([120 230 180]+128)/(256+128);patch([0 1 1 0],[0 0 1 1],c1);patch([0 1 1 1-e 1-e 0+e],[0 0 1 1-e 0+e 0+e],c2);patch([0 0 1 1-e 0+e 0+e],[0 1 1 1-e 1-e 0+e],c3);plot([0 1 1 0 0],[0 0 1 1 0]);
  wires:
  "p{2}"/1 -> mux/1
  mux/1 -> "pd{2,1}"/1
